simulink model "VelocityIntegratorTest"  (R2016a)
settings: Solver=VariableStepAuto  StartTime=0.0  StopTime=100  RelTol=1e-3
libraries: SimscapeMacros x4, fl_lib x1, nesl_utility x1, ProjectBlocks x1
settings Model: Creator=Peter  LastModifiedBy=Peter

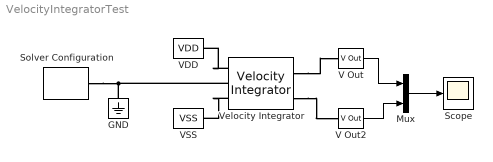
== system VelocityIntegratorTest ==
  GND : fl_lib/Electrical/Electrical Elements/Electrical Reference
  Mux : Mux  Inputs=2
  Scope : Scope
  Solver Configuration : nesl_utility/Solver Configuration  PhysicalDomain=network_engine_domain  SubClassName=solver  LeftPortType=input  RightPortType=generic  Accelerate=off  Tones=[]  Harmonics=[]  SimulateNoise=off  Profile=off  UseLocalSampling=off  EnableSwitchedLinearOptims=on  FrequencyDomain=off  UseCCode=off  RelTol=0.001  AbsTol=1e-06  MinStep=1e-09  ToWorkspace=off  RevertToSquareIcSolve=off  NumHomotopyIterations=100  PhasorMode=off  PhasorModeNumHarmonics=1  OverrideAbsTol=off  DoDC=off  ResidualTolerance=1e-09  UseLocalSolver=off  LocalSolverChoice=NE_BACKWARD_EULER_ADVANCER  LocalSolverSampleTime=0.001  DoFixedCost=off  MaxNonlinIter=3  MaxModeIter=2  LinearAlgebra=Sparse  DelaysMemoryBudget=1024  AutomaticFiltering=on  FilteringTimeConstant=0.001
  V Out : SimscapeMacros/V Out
  V Out2 : SimscapeMacros/V Out
  VDD : SimscapeMacros/VDD
  VSS : SimscapeMacros/VSS
  Velocity Integrator : ProjectBlocks/Velocity Integrator
  wires:
  Mux/1 -> Scope/1
  V Out/1 -> Mux/1
  V Out2/1 -> Mux/2
  connections:
  Solver Configuration/RConn1 -- Velocity Integrator/LConn2 -- GND/LConn1
  Velocity Integrator/LConn1 -- VDD/RConn1
  Velocity Integrator/RConn1 -- V Out/LConn1
  Velocity Integrator/RConn2 -- V Out2/LConn1
  Velocity Integrator/LConn3 -- VSS/RConn1
